simulink model "T1"  (R2018a)
settings: Solver=VariableStepAuto  StartTime=0.0  StopTime=10.0  RelTol=1e-3
values from neighbouring files (symbols this model uses):
  B = 0.1    [AT1.m]
  didt0 = (-R/L)*i0-(Kw/L)*w0+(1/L)*V0    (= 0)    [AT1.m]
  dwdt0 = (-B/J)*w0-(1/J)*Tc0+(5.26/J)*exp(-i0)    [AT1.m]
  i0 = 0    [AT1.m]
  J = 1    [AT1.m]
  Kw = 1/3    (= 0.333333333333)    [AT1.m]
  L = 0.5    [AT1.m]
  R = 10    [AT1.m]
  Tc0 = 0    [AT1.m]
  V0 = 0    [AT1.m]
  w0 = 0    [AT1.m]
settings Model: Creator=VanderleiMunhozPerei  LastModifiedBy=VanderleiMunhozPerei

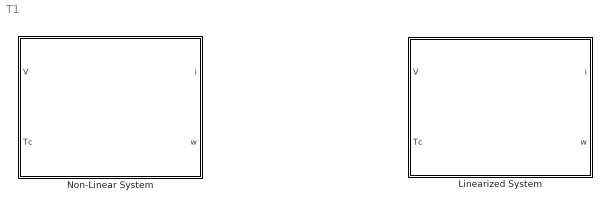
== system T1 ==
  Linearized System : Subsystem
  Non-Linear System : Subsystem

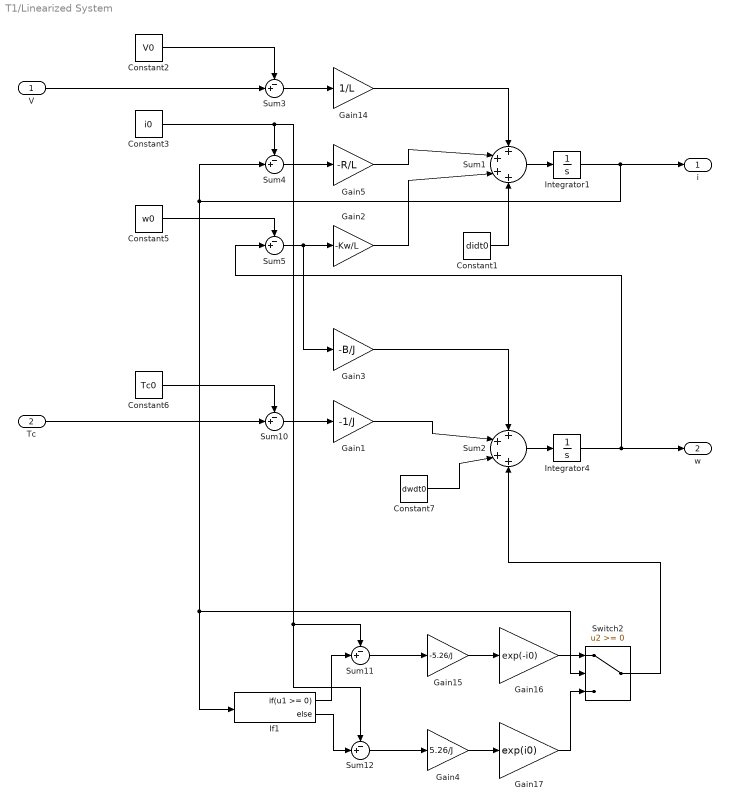
== system T1/Linearized System ==
  V : Inport
  Tc : Inport  Port=2
  Constant1 : Constant  Value=didt0
  Constant2 : Constant  Value=V0
  Constant3 : Constant  Value=i0
  Constant5 : Constant  Value=w0
  Constant6 : Constant  Value=Tc0
  Constant7 : Constant  Value=dwdt0
  Gain1 : Gain  Gain=-1/J
  Gain14 : Gain  Gain=1/L
  Gain15 : Gain  Gain=-5.26/J
  Gain16 : Gain  Gain=exp(-i0)
  Gain17 : Gain  Gain=exp(i0)
  Gain2 : Gain  Gain=-Kw/L
  Gain3 : Gain  Gain=-B/J
  Gain4 : Gain  Gain=5.26/J
  Gain5 : Gain  Gain=-R/L
  If1 : If  IfExpression=u1 >= 0
  Integrator1 : Integrator
  Integrator4 : Integrator
  Sum1 : Sum  Inputs=+|+|+|+
  Sum{3..5,10..12} (6 alike) : Sum  Inputs=-+|
  Sum2 : Sum  Inputs=+|+|+|+
  Switch2 : Switch
  i : Outport
  w : Outport  Port=2
  wires:
  Gain17/1 -> Switch2/3
  Sum5/1 -> Gain3/1, Gain2/1
  Integrator1/1 -> i/1, If1/1, Switch2/2, Sum4/2
  Sum4/1 -> Gain5/1
  Sum11/1 -> Gain15/1
  Sum1/1 -> Integrator1/1
  Gain5/1 -> Sum1/2
  Gain2/1 -> Sum1/3
  Tc/1 -> Sum10/2
  Sum3/1 -> Gain14/1
  Constant3/1 -> Sum11/1, Sum12/1, Sum4/1
  Constant2/1 -> Sum3/1
  Gain3/1 -> Sum2/1
  Integrator4/1 -> w/1, Sum5/2
  Constant5/1 -> Sum5/1
  Sum10/1 -> Gain1/1
  Gain16/1 -> Switch2/1
  Gain14/1 -> Sum1/1
  Gain1/1 -> Sum2/2
  If1/1 -> Sum11/2
  If1/2 -> Sum12/2
  Constant6/1 -> Sum10/1
  Sum2/1 -> Integrator4/1
  V/1 -> Sum3/2
  Switch2/1 -> Sum2/4
  Sum12/1 -> Gain4/1
  Gain4/1 -> Gain17/1
  Constant7/1 -> Sum2/3
  Gain15/1 -> Gain16/1
  Constant1/1 -> Sum1/4

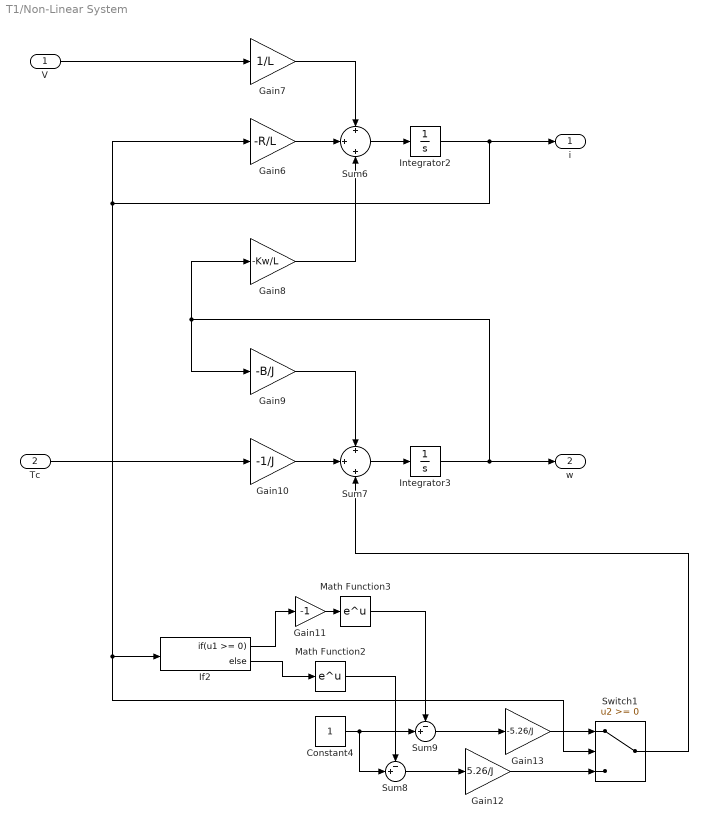
== system T1/Non-Linear System ==
  V : Inport
  Tc : Inport  Port=2
  Constant4 : Constant
  Gain10 : Gain  Gain=-1/J
  Gain11 : Gain  Gain=-1
  Gain12 : Gain  Gain=5.26/J
  Gain13 : Gain  Gain=-5.26/J
  Gain6 : Gain  Gain=-R/L
  Gain7 : Gain  Gain=1/L
  Gain8 : Gain  Gain=-Kw/L
  Gain9 : Gain  Gain=-B/J
  If2 : If  IfExpression=u1 >= 0
  Integrator2 : Integrator
  Integrator3 : Integrator
  Math Function2 : Math  SaturateOnIntegerOverflow=on
  Math Function3 : Math  SaturateOnIntegerOverflow=on
  Sum6 : Sum  Inputs=+|+|+
  Sum7 : Sum  Inputs=+|+|+
  Sum8 : Sum  Inputs=-+|
  Sum9 : Sum  Inputs=-+|
  Switch1 : Switch
  i : Outport
  w : Outport  Port=2
  wires:
  Sum7/1 -> Integrator3/1
  Sum6/1 -> Integrator2/1
  Integrator3/1 -> w/1, Gain9/1, Gain8/1
  If2/2 -> Math Function2/1
  Sum8/1 -> Gain12/1
  Gain11/1 -> Math Function3/1
  Gain7/1 -> Sum6/1
  Integrator2/1 -> i/1, Gain6/1, If2/1, Switch1/2
  Gain9/1 -> Sum7/1
  Gain10/1 -> Sum7/2
  Switch1/1 -> Sum7/3
  Gain13/1 -> Switch1/1
  Gain8/1 -> Sum6/3
  Sum9/1 -> Gain13/1
  V/1 -> Gain7/1
  Constant4/1 -> Sum9/2, Sum8/2
  Math Function2/1 -> Sum8/1
  Math Function3/1 -> Sum9/1
  If2/1 -> Gain11/1
  Gain6/1 -> Sum6/2
  Gain12/1 -> Switch1/3
  Tc/1 -> Gain10/1
